simulink model "LR_1_var2"  (R2020b)
settings: Solver=FixedStepAuto  StartTime=0.0  StopTime=5  FixedStep=0.00001  RelTol=1e-3
values from neighbouring files (symbols this model uses):
  A = 6    [Param_LR_1_var2.m]
  a = 3    [Param_LR_1_var2.m]
  delta = 0.6    [Param_LR_1_var2.m]
  k = 5    [Param_LR_1_var2.m]
libraries: simulink x5
settings Model: Creator=SIA  LastModifiedBy=SIA
settings SolverCC: ZeroCrossAlgorithm=Adaptive
settings DebuggingCC: IgnoredZcDiagnostic=none

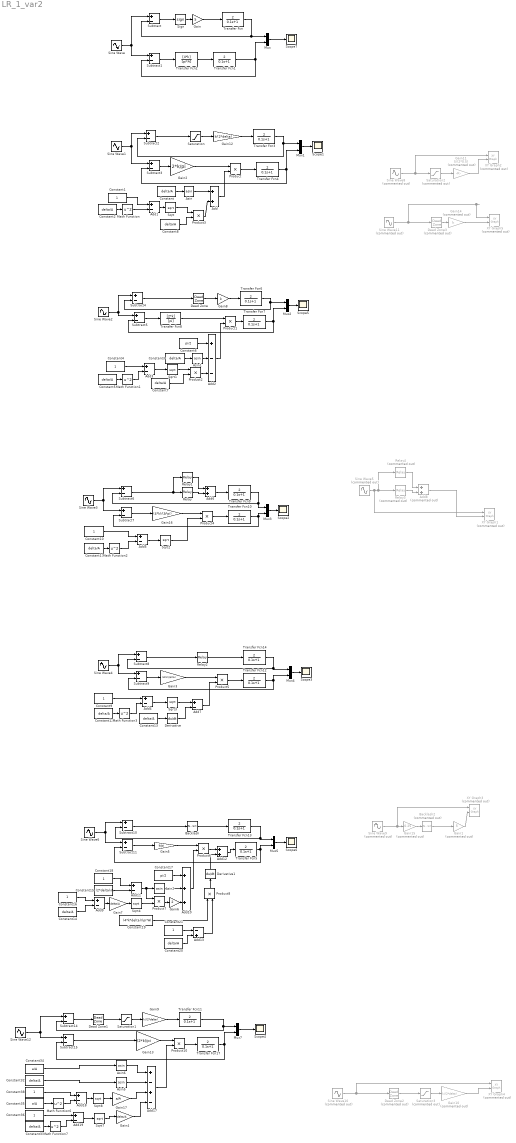
== system LR_1_var2 ==
  Add : Sum
  Add{1,3..5,7,9,11,18..19} (9 alike) : Sum  Inputs=+-
  Add10 : Sum  Inputs=+++
  Add12 : Sum
  Add13 : Sum  Inputs=-+
  Add17 : Sum  Inputs=+-+-
  Add2 : Sum  Inputs=+--
  Add6 : Sum
  Add8 : Sum  Commented=on
  Asin{,1..2,5..6} (5 alike) : Trigonometry  Operator=asin
  Backlash : Backlash  BacklashWidth=delta
  Backlash2 : Backlash  Commented=on
  Constant{,2..3,5,7..8,11..14,20,32..33} (13 alike) : Constant  Value=delta/A
  Constant{1,4,9..10,16,18,21,36,38} (9 alike) : Constant
  Constant15 : Constant  Value=(2*delta)/A
  Constant17 : Constant  Value=pi/2
  Constant19 : Constant  Value=(4*k*delta)/(pi*A)
  Constant34 : Constant  Value=a/A
  Constant35 : Constant  Value=a/A
  Constant6 : Constant  Value=pi/2
  Dead Zone : DeadZone  LowerValue=-delta  UpperValue=delta  SaturateOnIntegerOverflow=on
  Dead Zone1 : DeadZone  LowerValue=-delta  UpperValue=delta  SaturateOnIntegerOverflow=on
  Dead Zone2 : DeadZone  Commented=on  LowerValue=-delta  UpperValue=delta  SaturateOnIntegerOverflow=on
  Dead Zone3 : DeadZone  Commented=on  LowerValue=-delta  UpperValue=delta  SaturateOnIntegerOverflow=on
  Derivative : Derivative
  Derivative1 : Derivative
  Gain : Gain  Gain=5
  Gain1 : Gain  Commented=on  Gain=5
  Gain10 : Gain  Commented=on  Gain=k/(2*delta)
  Gain11 : Gain  Commented=on  Gain=5/(2*0.5)
  Gain12 : Gain  Gain=k/(2*delta)
  Gain13 : Gain  Gain=(2*k)/pi
  Gain14 : Gain  Commented=on  Gain=k
  Gain15 : Gain  Commented=on  Gain=0.25
  Gain16 : Gain  Gain=(4*k)/(A*pi)
  Gain17 : Gain  Gain=a/A
  Gain2 : Gain  Gain=2*k/pi
  Gain3 : Gain  Gain=(4*k)/(pi*A)
  Gain4 : Gain  Gain=delta/A
  Gain5 : Gain  Gain=k/pi
  Gain6 : Gain  Gain=2
  Gain7 : Gain  Gain=delta/A
  Gain8 : Gain  Gain=k
  Gain9 : Gain  Gain=k/(2*delta)
  Math Function{,1..3,6..7} (6 alike) : Math  Operator=square  SaturateOnIntegerOverflow=on
  Mux{,1..5,7} (7 alike) : Mux  Inputs=2
  Product{,1..8,10} (10 alike) : Product
  Relay : Relay  OnSwitchValue=-delta  OffSwitchValue=-delta  OnOutputValue=0  OffOutputValue=-k
  Relay1 : Relay  OnSwitchValue=delta  OffSwitchValue=delta  OnOutputValue=k
  Relay2 : Relay  OnSwitchValue=delta  OffSwitchValue=-delta  OnOutputValue=k  OffOutputValue=-k
  Relay3 : Relay  Commented=on  OnSwitchValue=-0.5  OffSwitchValue=-0.5  OnOutputValue=0  OffOutputValue=-1
  Relay4 : Relay  Commented=on  OnSwitchValue=0.5  OffSwitchValue=0.5
  Saturation : Saturate  UpperLimit=delta  LowerLimit=-delta
  Saturation1 : Saturate  UpperLimit=a-delta  LowerLimit=-(a-delta)
  Saturation2 : Saturate  Commented=on
  Saturation3 : Saturate  Commented=on  UpperLimit=a-delta  LowerLimit=-(a-delta)
  Scope{1..7} (7 alike) : Scope
  Sign : Signum
  Sine Wave : Sin  Frequency=5  SampleTime=0
  Sine Wave{1..4,6,12} (6 alike) : Sin  Amplitude=A  Frequency=5  SampleTime=0
  Sine Wave10 : Sin  Commented=on  Amplitude=6  Frequency=5  SampleTime=0.01
  Sine Wave11 : Sin  Commented=on  Amplitude=3  Frequency=5  SampleTime=0.01
  Sine Wave5 : Sin  Commented=on  Amplitude=5  Frequency=5  SampleTime=0
  Sine Wave8 : Sin  Commented=on  Amplitude=3  Frequency=5  SampleTime=0.01
  Sine Wave9 : Sin  Commented=on  Amplitude=15  Frequency=5  SampleTime=0.01
  Sqrt{,1..4,7..8} (7 alike) : Sqrt  SaturateOnIntegerOverflow=on
  Subtract{,1..11,14..15} (14 alike) : Sum  Inputs=+-
  Transfer Fcn{,1,3..7,9..14,17} (14 alike) : TransferFcn  Numerator=[2]  Denominator=[0.1 1]
  Transfer Fcn2 : TransferFcn  Numerator=[4*k]  Denominator=[pi*A]
  Transfer Fcn8 : TransferFcn  Numerator=[2*k]  Denominator=[pi]
  XY Graph1 : simulink/Sinks/XY Graph  Commented=on  xmin=-1.5  xmax=1.5  ymin=-1.5  ymax=1.5  st=0.0001
  XY Graph2 : simulink/Sinks/XY Graph  Commented=on  xmin=-3  xmax=3  ymin=-5  ymax=5  st=-1
  XY Graph3 : simulink/Sinks/XY Graph  Commented=on  xmin=-10  xmax=10  ymin=-8  ymax=8  st=0.11
  XY Graph4 : simulink/Sinks/XY Graph  Commented=on  xmin=-3  xmax=3  ymin=-8  ymax=8  st=0.01
  XY Graph5 : simulink/Sinks/XY Graph  Commented=on  xmin=-2  xmax=2  ymin=-1  ymax=1  st=-1
  wires:
  Sine Wave/1 -> Subtract1/1, Subtract/1
  Mux/1 -> Scope7/1
  Transfer Fcn/1 -> Subtract/2, Mux/1
  Transfer Fcn1/1 -> Mux/2, Subtract1/2
  Subtract/1 -> Sign/1
  Sign/1 -> Gain/1
  Gain/1 -> Transfer Fcn/1
  Subtract1/1 -> Transfer Fcn2/1
  Transfer Fcn2/1 -> Transfer Fcn1/1
  Sine Wave1/1 -> Subtract3/1, Subtract2/1
  Subtract3/1 -> Gain2/1
  Transfer Fcn4/1 -> Mux1/2, Subtract3/2
  Product/1 -> Transfer Fcn4/1
  Transfer Fcn3/1 -> Subtract2/2, Mux1/1
  Mux1/1 -> Scope1/1
  Constant/1 -> Asin/1
  Add/1 -> Product/2
  Gain2/1 -> Product/1
  Asin/1 -> Add/1
  Constant1/1 -> Add1/1
  Add1/1 -> Sqrt/1
  Math Function/1 -> Add1/2
  Constant2/1 -> Math Function/1
  Mux2/1 -> Scope5/1
  Math Function1/1 -> Add3/2
  Add3/1 -> Sqrt1/1
  Constant4/1 -> Add3/1
  Constant5/1 -> Math Function1/1
  Sine Wave2/1 -> Subtract5/1, Subtract4/1
  Subtract5/1 -> Transfer Fcn8/1
  Transfer Fcn8/1 -> Product1/1
  Constant3/1 -> Asin1/1
  Transfer Fcn7/1 -> Mux2/2, Subtract5/2
  Add2/1 -> Product1/2
  Transfer Fcn6/1 -> Subtract4/2, Mux2/1
  Subtract4/1 -> Dead Zone/1
  Product1/1 -> Transfer Fcn7/1
  Asin1/1 -> Add2/2
  Constant6/1 -> Add2/1
  Product2/1 -> Add2/3
  Sqrt1/1 -> Product2/1
  Constant7/1 -> Product2/2
  Product3/1 -> Add/2
  Sqrt/1 -> Product3/1
  Constant8/1 -> Product3/2
  Subtract6/1 -> Relay1/1, Relay/1
  Product4/1 -> Transfer Fcn10/1
  Sqrt2/1 -> Product4/2
  Transfer Fcn9/1 -> Mux3/1, Subtract6/2
  Transfer Fcn10/1 -> Mux3/2, Subtract7/2
  Gain16/1 -> Product4/1
  Subtract7/1 -> Gain16/1
  Sine Wave3/1 -> Subtract7/1, Subtract6/1
  Constant10/1 -> Add5/1
  Math Function2/1 -> Add5/2
  Constant11/1 -> Math Function2/1
  Mux3/1 -> Scope2/1
  Add5/1 -> Sqrt2/1
  Add6/1 -> Transfer Fcn9/1
  Relay1/1 -> Add6/1
  Relay/1 -> Add6/2
  Mux4/1 -> Scope3/1
  Math Function3/1 -> Add4/2
  Constant12/1 -> Math Function3/1
  Add4/1 -> Sqrt3/1
  Sine Wave4/1 -> Subtract9/1, Subtract8/1
  Constant9/1 -> Add4/1
  Subtract9/1 -> Gain3/1
  Gain3/1 -> Product5/1
  Transfer Fcn12/1 -> Mux4/2, Subtract9/2
  Transfer Fcn14/1 -> Mux4/1, Subtract8/2
  Relay2/1 -> Transfer Fcn14/1
  Product5/1 -> Transfer Fcn12/1
  Subtract8/1 -> Relay2/1
  Sqrt3/1 -> Add7/1
  Constant13/1 -> Derivative/1
  Add7/1 -> Product5/2
  Relay4/1 -> Add8/1
  Relay3/1 -> Add8/2
  Sine Wave5/1 -> XY Graph1/1, Relay4/1, Relay3/1
  Add8/1 -> XY Graph1/2
  Gain5/1 -> Product6/1
  Transfer Fcn13/1 -> Mux5/1, Subtract10/2
  Transfer Fcn5/1 -> Mux5/2, Subtract11/2
  Constant16/1 -> Add9/1
  Constant14/1 -> Add9/2
  Add9/1 -> Gain7/1
  Mux5/1 -> Scope6/1
  Subtract11/1 -> Gain5/1
  Add10/1 -> Product6/2
  Sine Wave6/1 -> Subtract11/1, Subtract10/1
  Constant17/1 -> Add10/1
  Asin2/1 -> Add10/2
  Constant15/1 -> Add11/2
  Constant18/1 -> Add11/1
  Add11/1 -> Product7/1, Asin2/1
  Gain6/1 -> Add10/3
  Product7/1 -> Gain6/1
  Sqrt4/1 -> Product7/2
  Gain7/1 -> Sqrt4/1
  Product6/1 -> Add12/1
  Add12/1 -> Transfer Fcn5/1
  Product8/1 -> Derivative1/1
  Constant19/1 -> Product8/1
  Constant20/1 -> Add13/2
  Constant21/1 -> Add13/1
  Add13/1 -> Product8/2
  Saturation/1 -> Gain12/1
  Sine Wave8/1 -> Saturation2/1, XY Graph2/1
  Subtract2/1 -> Saturation/1
  Gain15/1 -> Backlash2/1
  Sine Wave9/1 -> Gain15/1, XY Graph3/1
  Gain1/1 -> XY Graph3/2
  Backlash2/1 -> Gain1/1
  Gain10/1 -> XY Graph4/2
  Saturation2/1 -> Gain11/1
  Gain11/1 -> XY Graph2/2
  Gain12/1 -> Transfer Fcn3/1
  Dead Zone3/1 -> Gain14/1
  Sine Wave11/1 -> Dead Zone3/1, XY Graph5/1
  Subtract10/1 -> Backlash/1
  Backlash/1 -> Transfer Fcn13/1
  Gain14/1 -> XY Graph5/2
  Dead Zone/1 -> Gain8/1
  Derivative/1 -> Add7/2
  Derivative1/1 -> Add12/2
  Saturation1/1 -> Gain9/1
  Add19/1 -> Sqrt7/1
  Add17/1 -> Product10/2
  Asin6/1 -> Add17/1
  Constant36/1 -> Add19/1
  Asin5/1 -> Add17/2
  Gain4/1 -> Add17/4
  Constant33/1 -> Math Function7/1
  Math Function7/1 -> Add19/2
  Sqrt7/1 -> Gain4/1
  Sqrt8/1 -> Gain17/1
  Math Function6/1 -> Add18/2
  Constant35/1 -> Math Function6/1
  Add18/1 -> Sqrt8/1
  Transfer Fcn17/1 -> Subtract15/2, Mux7/2
  Gain17/1 -> Add17/3
  Product10/1 -> Transfer Fcn17/1
  Constant32/1 -> Asin5/1
  Sine Wave12/1 -> Subtract15/1, Subtract14/1
  Gain13/1 -> Product10/1
  Constant34/1 -> Asin6/1
  Constant38/1 -> Add18/1
  Mux7/1 -> Scope4/1
  Transfer Fcn11/1 -> Subtract14/2, Mux7/1
  Subtract15/1 -> Gain13/1
  Dead Zone1/1 -> Saturation1/1
  Subtract14/1 -> Dead Zone1/1
  Gain8/1 -> Transfer Fcn6/1
  Gain9/1 -> Transfer Fcn11/1
  Sine Wave10/1 -> Dead Zone2/1, XY Graph4/1
  Saturation3/1 -> Gain10/1
  Dead Zone2/1 -> Saturation3/1
